simulink library "NeuroMuscularLibrary"  (R2019a)
settings: Solver=ode45  StartTime=0.0  StopTime=10.0  RelTol=1e-3  EnableMultiTasking=on
undefined symbols (not defined in the file): a2loptHAB, a2loptHAD, a2loptHAMsw, a2loptRFsw, ankle_height, aRefHAB, aRefHAD, aRefHAMsw, aRefRFsw, c, c_jointstop, deltaLegAngleThr, DeltaThRef, eref, Fmax, FmaxGLU, footBallToAnkleDist, footBallToCGDist, footBallToCGDist_y, footBallToHeelDist, footCenterlineToBall, footCenterlineToHeel, footInertia, footLength, footMass, FT, FT_GLU, GainDphiHATGLUst, GainDphiHATHABst, GainDphiHATHADst, GainDphiHATHFLst, GainFGASst, GainFGLUst, GainFHABst, GainFHAMst, GainFSOLst, GainFSOLTAst, GainFVASst, GainLBFSHst, GainLBFSHVASst, GainLGLUsw, GainLHABsw, GainLHADsw, GainLHAMGLUsw, GainLHAMsw, GainLRFHFLsw, GainLTAst, GainLTAsw, GainLVASsw, GainPhiHATGLUst, GainPhiHATHABst, GainPhiHATHADst, GainPhiHATHFLst, GainSGLUcHFLst, GainSGLUHAMst, GainSHABcHABst, GainSHADcHADst, GainSHAMBFSHsw, GainSHAMcHFLst, GainSHAMGASsw ... (+175)
libraries: sm_lib x54, $bdroot x45, nesl_utility x39, simulink x24, simulink_extras x6, vrlib x5, dspsigops x4
(part 3 of 5)

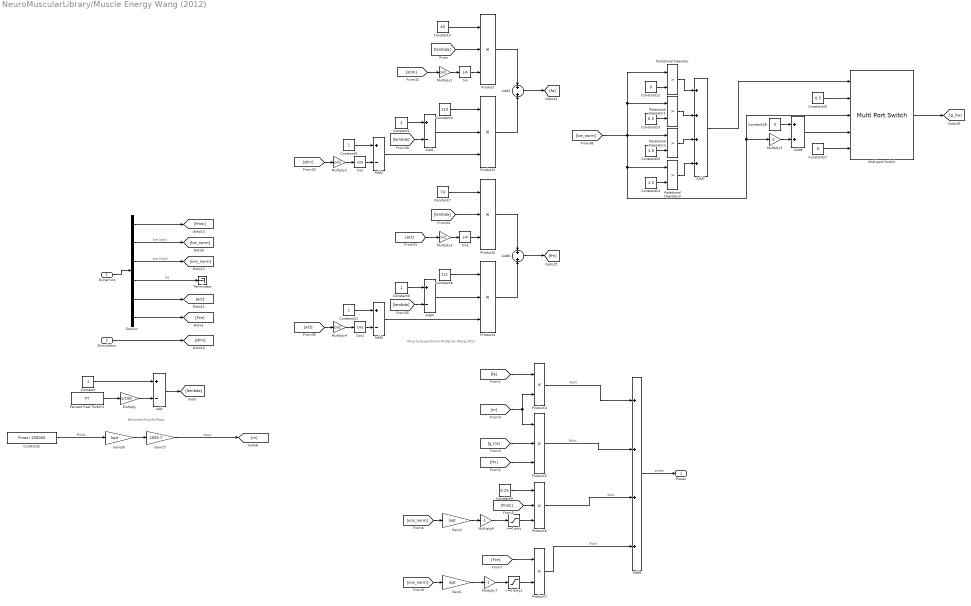
== system NeuroMuscularLibrary/Muscle Energy Wang (2012) ==
  note: Muscle Expenditure Model by Wang 2012
  note: Estimate Muscle Mass
  Dynamics : Inport
  Stimulation : Inport  Port=2
  >=0 only : Saturate  UpperLimit=inf  LowerLimit=0  ZeroCross=off
  >=0 only1 : Saturate  UpperLimit=inf  LowerLimit=0  ZeroCross=off
  Add{,1..2,4..5} (5 alike) : Sum  Inputs=+-
  Add3 : Sum
  Add6 : Sum
  Add7 : Sum  Inputs=++++
  Add8 : Sum
  Add9 : Sum  Inputs=++++
  Constant{,1,5..6,11} (5 alike) : Constant
  Constant12 : Constant  Value=0
  Constant2 : Constant  Value=Fmax/ 250000
  Constant23 : Constant  Value=0.5
  Constant24 : Constant  Value=1.5
  Constant25 : Constant  Value=1.0
  Constant26 : Constant  Value=0.5
  Constant27 : Constant  Value=0
  Constant28 : Constant  Value=3
  Constant3 : Constant  Value=40
  Constant4 : Constant  Value=133
  Constant7 : Constant  Value=74
  Constant8 : Constant  Value=111
  Constant9 : Constant  Value=0.25
  Cos : Trigonometry  Operator=cos
  Cos1 : Trigonometry  Operator=cos
  Demux : Demux  Outputs=6
  Gain1 : Gain  Gain=lopt
  Gain2 : Gain  Gain=lopt
  Gain26 : Gain  Gain=lopt
  Gain27 : Gain  Gain=1059.7
  Multiply : Gain  Gain=1/100
  Multiply{1..4} (4 alike) : Gain  Gain=pi/2
  Multiply5 : Gain  Gain=-2
  Multiply6 : Gain  Gain=-1
  Multiply7 : Gain  Gain=-1
  Multiport Switch : MultiPortSwitch  Inputs=4  DiagnosticForDefault=Warning
  Percent Fast Twitch1 : Constant  Value=FT
  Product{,1..3,5..6} (6 alike) : Product  Inputs=3
  Product4 : Product
  Product7 : Product
  Relational Operator{,1..3} (4 alike) : RelationalOperator  Operator=>  OutDataTypeStr=boolean  RndMeth=Simplest
  Sin : Trigonometry
  Sin1 : Trigonometry
  Terminator : Terminator
  Power : Outport  VectorParamsAs1DForOutWhenUnconnected=on
  wires:
  Demux/6 -> [Fce]
  [vce_norm] -> Gain1/1
  Product7/1 -> Add9/4  "Wdot"
  [Fce] -> Product7/1
  Multiply7/1 -> >=0 only1/1
  Product6/1 -> Add9/3  "Sdot"
  Multiply6/1 -> >=0 only/1
  [vce_norm] -> Gain2/1
  Constant9/1 -> Product6/1
  [Fmtc] -> Product6/2
  Product5/1 -> Add9/2  "Mdot"
  Product4/1 -> Add9/1  "Adot"
  [fm] -> Product5/3
  [g_lce] -> Product5/2
  [fa] -> Product4/1
  [m] -> Product4/2, Product5/1
  Constant2/1 -> Gain26/1  "PCSAL"
  Gain27/1 -> [m]  "Mass"
  Gain26/1 -> Gain27/1
  Multiply5/1 -> Add8/2
  Constant28/1 -> Add8/1
  Add8/1 -> Multiport Switch/4
  Constant27/1 -> Multiport Switch/5
  Constant26/1 -> Multiport Switch/2
  Add7/1 -> Multiport Switch/1
  Relational Operator3/1 -> Add7/4
  Relational Operator2/1 -> Add7/3
  Relational Operator1/1 -> Add7/2
  Relational Operator/1 -> Add7/1
  Constant24/1 -> Relational Operator3/2
  Constant25/1 -> Relational Operator2/2
  Constant23/1 -> Relational Operator1/2
  Constant12/1 -> Relational Operator/2
  [lce_norm] -> Multiport Switch/3, Multiply5/1, Relational Operator3/1, Relational Operator1/1, Relational Operator/1, Relational Operator2/1
  Constant7/1 -> Product2/1
  [act] -> Multiply3/1
  [act] -> Multiply4/1
  [lambda] -> Add4/2
  Cos1/1 -> Add5/2
  Multiply4/1 -> Cos1/1
  Add6/1 -> [fm]
  Constant8/1 -> Product3/1
  [lambda] -> Product2/2
  Add5/1 -> Product3/3
  Add4/1 -> Product3/2
  Multiply3/1 -> Sin1/1
  Constant6/1 -> Add4/1
  Sin1/1 -> Product2/3
  Product2/1 -> Add6/1
  Product3/1 -> Add6/2
  Constant11/1 -> Add5/1
  Cos/1 -> Add2/2
  Add3/1 -> [fa]
  Product/1 -> Add3/1
  Product1/1 -> Add3/2
  Multiply2/1 -> Cos/1
  [stim] -> Multiply2/1
  [stim] -> Multiply1/1
  Multiply1/1 -> Sin/1
  Sin/1 -> Product/3
  Constant5/1 -> Add2/1
  Add2/1 -> Product1/3
  Constant4/1 -> Product1/1
  Add1/1 -> Product1/2
  Constant3/1 -> Product/1
  Constant1/1 -> Add1/1
  [lambda] -> Add1/2
  [lambda] -> Product/2
  Add/1 -> [lambda]
  Multiply/1 -> Add/2
  Percent Fast Twitch1/1 -> Multiply/1
  Constant/1 -> Add/1
  Add9/1 -> Power/1  "power"
  Dynamics/1 -> Demux/1
  Stimulation/1 -> [stim]
  Demux/1 -> [Fmtc]
  Demux/3 -> [vce_norm]  "vce [lopt]"
  Demux/5 -> [act]
  Demux/4 -> Terminator/1  "lse"
  Demux/2 -> [lce_norm]  "lce [opt]"
  >=0 only/1 -> Product6/3
  >=0 only1/1 -> Product7/2
  Multiport Switch/1 -> [g_lce]
  Gain1/1 -> Multiply7/1
  Gain2/1 -> Multiply6/1

== system NeuroMuscularLibrary/Norm ==
  Vector : Inport
  Add4 : Sum  Inputs=+
  Square : Math  Operator=square  SaturateOnIntegerOverflow=on
  Square Root : Sqrt  SaturateOnIntegerOverflow=on
  Norm : Outport  VectorParamsAs1DForOutWhenUnconnected=on
  wires:
  Add4/1 -> Square Root/1
  Square/1 -> Add4/1
  Vector/1 -> Square/1
  Square Root/1 -> Norm/1

== system NeuroMuscularLibrary/Overextension Joint Limit ==
  note: Knee/Hip Joint Limits
  phi [rad] : Inport
  dphi [rad/s] : Inport  Port=2
  Gain1 : Gain  Gain=ext
  Gain2 : Gain  Gain=-ext
  Gain3 : Gain  Gain=c_jointstop
  Gain4 : Gain  Gain=1/w_max_jointstop
  Gain5 : Gain  Gain=ext
  Limit Ankle Range : simulink/Logic and Bit Operations/Interval Test  Commented=on  IntervalClosedRight=on  uplimit=185*pi/180  IntervalClosedLeft=on  lowlimit=40*pi/180  OutDataTypeStr=boolean
  Logical Operator3 : Logic  Commented=on  Operator=NOT  AllPortsSameDT=off  OutDataTypeStr=boolean
  Mux3 : Mux  Inputs=2
  Overextension Torque : Fcn  Expr="- u(1)  *  (1-u(2)) * (u(2)<1) * (u(1)>0)"
  Stop Simulation1 : Stop  Commented=on
  Sum : Sum  Inputs=|+-
  overextension angle : Constant  Value=phiUpLimit
  M_stop [Nm] : Outport  VectorParamsAs1DForOutWhenUnconnected=on
  wires:
  Gain5/1 -> M_stop [Nm]/1
  Overextension Torque/1 -> Gain5/1
  Logical Operator3/1 -> Stop Simulation1/1
  Limit Ankle Range/1 -> Logical Operator3/1
  Gain2/1 -> Mux3/2
  Gain4/1 -> Gain2/1
  Sum/1 -> Gain3/1
  phi [rad]/1 -> Limit Ankle Range/1, Sum/1
  overextension angle/1 -> Sum/2
  dphi [rad/s]/1 -> Gain4/1
  Mux3/1 -> Overextension Torque/1
  Gain3/1 -> Gain1/1
  Gain1/1 -> Mux3/1

== system NeuroMuscularLibrary/Overextension//Overflexion Joint Limit ==
  note: Overextension/Overflexion Joint Limit
  phi [rad] : Inport
  dphi [rad/s] : Inport  Port=2
  Gain1 : Gain  Gain=c_jointstop
  Gain2 : Gain  Gain=-1
  Gain3 : Gain  Gain=c_jointstop
  Gain4 : Gain  Gain=1/w_max_jointstop
  Limit Range : simulink/Logic and Bit Operations/Interval Test  Commented=on  IntervalClosedRight=on  uplimit=phi12_UpLimit + 40*pi/180  IntervalClosedLeft=on  lowlimit=phi12_LowLimit - 40*pi/180  OutDataTypeStr=boolean
  Logical Operator3 : Logic  Commented=on  Operator=NOT  AllPortsSameDT=off  OutDataTypeStr=boolean
  Mux1 : Mux  Inputs=2
  Mux3 : Mux  Inputs=2
  Overextension Torque : Fcn  Expr="- u(1)  *  (1-u(2)) * (u(2)<1) * (u(1)>0)"
  Overflexion Torque : Fcn  Expr="- u(1)  *  (1-u(2)) * (u(2)<1) * (u(1)<0)"
  Stop Simulation1 : Stop  Commented=on
  Sum : Sum  Inputs=|+-
  Sum1 : Sum  Inputs=|+-
  Sum2 : Sum
  overextension angle : Constant  Value=phiUpLimit
  overflexion angle : Constant  Value=phiLowLimit
  M_stop [Nm] : Outport  VectorParamsAs1DForOutWhenUnconnected=on
  wires:
  Mux3/1 -> Overextension Torque/1
  Gain3/1 -> Mux3/1
  dphi [rad/s]/1 -> Gain4/1
  overextension angle/1 -> Sum/2
  phi [rad]/1 -> Sum/1, Sum1/1, Limit Range/1
  Sum/1 -> Gain3/1
  Gain4/1 -> Gain2/1, Mux1/2
  Gain1/1 -> Mux1/1
  Sum1/1 -> Gain1/1
  overflexion angle/1 -> Sum1/2
  Mux1/1 -> Overflexion Torque/1
  Sum2/1 -> M_stop [Nm]/1
  Gain2/1 -> Mux3/2
  Overflexion Torque/1 -> Sum2/2
  Overextension Torque/1 -> Sum2/1
  Limit Range/1 -> Logical Operator3/1
  Logical Operator3/1 -> Stop Simulation1/1

== system NeuroMuscularLibrary/Pos//Rot Sensor ==
  Gain2 : Gain  Gain=-1
  Mux : Mux  Inputs=3
  PS-Simulink Converter : nesl_utility/PS-Simulink Converter  PhysicalDomain=network_engine_domain  SubClassName=ps_output  LeftPortType=input  RightPortType=output  PseudoPeriodic=off  Frequencies=[]  Unit=m  AffineConversion=off
  PS-Simulink Converter1 : nesl_utility/PS-Simulink Converter  PhysicalDomain=network_engine_domain  SubClassName=ps_output  LeftPortType=input  RightPortType=output  PseudoPeriodic=off  Frequencies=[]  Unit=m  AffineConversion=off
  PS-Simulink Converter2 : nesl_utility/PS-Simulink Converter  PhysicalDomain=network_engine_domain  SubClassName=ps_output  LeftPortType=input  RightPortType=output  PseudoPeriodic=off  Frequencies=[]  Unit=m  AffineConversion=off
  PS-Simulink Converter3 : nesl_utility/PS-Simulink Converter  PhysicalDomain=network_engine_domain  SubClassName=ps_output  LeftPortType=input  RightPortType=output  PseudoPeriodic=off  Frequencies=[]  Unit=rad  AffineConversion=off
  PS-Simulink Converter4 : nesl_utility/PS-Simulink Converter  PhysicalDomain=network_engine_domain  SubClassName=ps_output  LeftPortType=input  RightPortType=output  PseudoPeriodic=off  Frequencies=[]  Unit=rad  AffineConversion=off
  Position Sensor : sm_lib/Frames and Transforms/Transform Sensor  MeasurementFrame=World  SenseAngle=on  SenseAxis=on  SenseAngle1=off  SenseAngle2=off  SenseAngle3=off  SenseQ=off  SenseR=off  SenseOmegaX=off  SenseOmegaY=off  SenseOmegaZ=off  SenseOmega1=off  SenseOmega2=off  SenseOmega3=off  SenseQDot=off  SenseRDot=off  SenseAlphaX=off  SenseAlphaY=off  SenseAlphaZ=off  SenseAlpha1=off  SenseAlpha2=off  SenseAlpha3=off  SenseQDDot=off  SenseRDDot=off  SenseX=on  SenseY=on  SenseZ=on  SenseRad=off  SenseAzim=off  SenseDist=off  SenseInc=off  SenseXDot=off  SenseYDot=off  SenseZDot=off  SenseRadDot=off  SenseAzimDot=off  SenseDistDot=off  SenseIncDot=off  SenseXDDot=off  SenseYDDot=off  SenseZDDot=off  SenseRadDDot=off  SenseAzimDDot=off  SenseDistDDot=off  SenseIncDDot=off
  Product : Product
  Selector : Selector  InputPortWidth=3  IndexOptions=Index vector (dialog)  Indices=[3]  OutputSizes=1
  Sign : Signum
  F : PMIOPort  Side=Left
  B : PMIOPort  Port=2  Side=Right
  Position : Outport  VectorParamsAs1DForOutWhenUnconnected=on
  Rotation : Outport  Port=2  VectorParamsAs1DForOutWhenUnconnected=on
  wires:
  PS-Simulink Converter1/1 -> Mux/2
  PS-Simulink Converter/1 -> Mux/1
  Mux/1 -> Position/1
  PS-Simulink Converter2/1 -> Mux/3
  PS-Simulink Converter4/1 -> Selector/1
  Selector/1 -> Sign/1
  PS-Simulink Converter3/1 -> Product/1
  Sign/1 -> Product/2
  Gain2/1 -> Rotation/1
  Product/1 -> Gain2/1
  connections:
  Position Sensor/RConn1 -- F/RConn1
  PS-Simulink Converter3/LConn1 -- Position Sensor/RConn2
  B/RConn1 -- Position Sensor/LConn1
  Position Sensor/RConn4 -- PS-Simulink Converter/LConn1
  PS-Simulink Converter1/LConn1 -- Position Sensor/RConn5
  PS-Simulink Converter2/LConn1 -- Position Sensor/RConn6
  PS-Simulink Converter4/LConn1 -- Position Sensor/RConn3

== system NeuroMuscularLibrary/Position Sensor ==
  Mux : Mux  Inputs=3
  PS-Simulink Converter : nesl_utility/PS-Simulink Converter  PhysicalDomain=network_engine_domain  SubClassName=ps_output  LeftPortType=input  RightPortType=output  PseudoPeriodic=off  Frequencies=[]  Unit=m  AffineConversion=off
  PS-Simulink Converter1 : nesl_utility/PS-Simulink Converter  PhysicalDomain=network_engine_domain  SubClassName=ps_output  LeftPortType=input  RightPortType=output  PseudoPeriodic=off  Frequencies=[]  Unit=m  AffineConversion=off
  PS-Simulink Converter2 : nesl_utility/PS-Simulink Converter  PhysicalDomain=network_engine_domain  SubClassName=ps_output  LeftPortType=input  RightPortType=output  PseudoPeriodic=off  Frequencies=[]  Unit=m  AffineConversion=off
  Position Sensor : sm_lib/Frames and Transforms/Transform Sensor  MeasurementFrame=World  SenseAngle=off  SenseAxis=off  SenseAngle1=off  SenseAngle2=off  SenseAngle3=off  SenseQ=off  SenseR=off  SenseOmegaX=off  SenseOmegaY=off  SenseOmegaZ=off  SenseOmega1=off  SenseOmega2=off  SenseOmega3=off  SenseQDot=off  SenseRDot=off  SenseAlphaX=off  SenseAlphaY=off  SenseAlphaZ=off  SenseAlpha1=off  SenseAlpha2=off  SenseAlpha3=off  SenseQDDot=off  SenseRDDot=off  SenseX=on  SenseY=on  SenseZ=on  SenseRad=off  SenseAzim=off  SenseDist=off  SenseInc=off  SenseXDot=off  SenseYDot=off  SenseZDot=off  SenseRadDot=off  SenseAzimDot=off  SenseDistDot=off  SenseIncDot=off  SenseXDDot=off  SenseYDDot=off  SenseZDDot=off  SenseRadDDot=off  SenseAzimDDot=off  SenseDistDDot=off  SenseIncDDot=off
  World Frame : sm_lib/Frames and Transforms/World Frame
  Frame : PMIOPort  Side=Left
  Position : Outport  VectorParamsAs1DForOutWhenUnconnected=on
  wires:
  PS-Simulink Converter2/1 -> Mux/3
  Mux/1 -> Position/1
  PS-Simulink Converter/1 -> Mux/1
  PS-Simulink Converter1/1 -> Mux/2
  connections:
  Position Sensor/RConn4 -- PS-Simulink Converter2/LConn1
  Position Sensor/RConn2 -- PS-Simulink Converter/LConn1
  Position Sensor/RConn1 -- Frame/RConn1
  Position Sensor/RConn3 -- PS-Simulink Converter1/LConn1
  Position Sensor/LConn1 -- World Frame/RConn1

== system NeuroMuscularLibrary/Position Velocity Sensor ==
  Mux : Mux  Inputs=6
  PS-Simulink Converter : nesl_utility/PS-Simulink Converter  PhysicalDomain=network_engine_domain  SubClassName=ps_output  LeftPortType=input  RightPortType=output  PseudoPeriodic=off  Frequencies=[]  Unit=m  AffineConversion=off
  PS-Simulink Converter1 : nesl_utility/PS-Simulink Converter  PhysicalDomain=network_engine_domain  SubClassName=ps_output  LeftPortType=input  RightPortType=output  PseudoPeriodic=off  Frequencies=[]  Unit=m  AffineConversion=off
  PS-Simulink Converter2 : nesl_utility/PS-Simulink Converter  PhysicalDomain=network_engine_domain  SubClassName=ps_output  LeftPortType=input  RightPortType=output  PseudoPeriodic=off  Frequencies=[]  Unit=m  AffineConversion=off
  PS-Simulink Converter3 : nesl_utility/PS-Simulink Converter  PhysicalDomain=network_engine_domain  SubClassName=ps_output  LeftPortType=input  RightPortType=output  PseudoPeriodic=off  Frequencies=[]  Unit=m/s  AffineConversion=off
  PS-Simulink Converter4 : nesl_utility/PS-Simulink Converter  PhysicalDomain=network_engine_domain  SubClassName=ps_output  LeftPortType=input  RightPortType=output  PseudoPeriodic=off  Frequencies=[]  Unit=m/s  AffineConversion=off
  PS-Simulink Converter5 : nesl_utility/PS-Simulink Converter  PhysicalDomain=network_engine_domain  SubClassName=ps_output  LeftPortType=input  RightPortType=output  PseudoPeriodic=off  Frequencies=[]  Unit=m/s  AffineConversion=off
  Position Sensor : sm_lib/Frames and Transforms/Transform Sensor  MeasurementFrame=World  SenseAngle=off  SenseAxis=off  SenseAngle1=off  SenseAngle2=off  SenseAngle3=off  SenseQ=off  SenseR=off  SenseOmegaX=off  SenseOmegaY=off  SenseOmegaZ=off  SenseOmega1=off  SenseOmega2=off  SenseOmega3=off  SenseQDot=off  SenseRDot=off  SenseAlphaX=off  SenseAlphaY=off  SenseAlphaZ=off  SenseAlpha1=off  SenseAlpha2=off  SenseAlpha3=off  SenseQDDot=off  SenseRDDot=off  SenseX=on  SenseY=on  SenseZ=on  SenseRad=off  SenseAzim=off  SenseDist=off  SenseInc=off  SenseXDot=on  SenseYDot=on  SenseZDot=on  SenseRadDot=off  SenseAzimDot=off  SenseDistDot=off  SenseIncDot=off  SenseXDDot=off  SenseYDDot=off  SenseZDDot=off  SenseRadDDot=off  SenseAzimDDot=off  SenseDistDDot=off  SenseIncDDot=off
  World Frame1 : sm_lib/Frames and Transforms/World Frame
  Frame : PMIOPort  Side=Left
  Position and Velocity : Outport  VectorParamsAs1DForOutWhenUnconnected=on
  wires:
  PS-Simulink Converter1/1 -> Mux/2
  PS-Simulink Converter/1 -> Mux/1
  Mux/1 -> Position and Velocity/1
  PS-Simulink Converter2/1 -> Mux/3
  PS-Simulink Converter3/1 -> Mux/4
  PS-Simulink Converter4/1 -> Mux/5
  PS-Simulink Converter5/1 -> Mux/6
  connections:
  Position Sensor/RConn3 -- PS-Simulink Converter1/LConn1
  Position Sensor/RConn1 -- Frame/RConn1
  Position Sensor/RConn2 -- PS-Simulink Converter/LConn1
  Position Sensor/RConn4 -- PS-Simulink Converter2/LConn1
  Position Sensor/LConn1 -- World Frame1/RConn1
  PS-Simulink Converter3/LConn1 -- Position Sensor/RConn5
  PS-Simulink Converter4/LConn1 -- Position Sensor/RConn6
  PS-Simulink Converter5/LConn1 -- Position Sensor/RConn7

== system NeuroMuscularLibrary/RF Link ==
  note: RF Attachment
  hip angle : Inport
  knee angle : Inport  Port=2
  Constant3 : Constant  Value=rRFh
  Constant4 : Constant  Value=lslackRF+loptRF
  Constant5 : Constant  Value=phirefRFh
  Constant6 : Constant  Value=phirefRFk
  Constant7 : Constant  Value=phimaxRFk  VectorParams1D=off
  Demux1 : Demux  Outputs=2
  Gain1 : Gain  Gain=phiScaleRFk
  Gain2 : Gain  Gain=rhoRFh
  Gain3 : Gain  Gain=rRFkmax
  Gain4 : Gain  Gain=rhoRFk/phiScaleRFk
  Gain5 : Gain  Gain=phiScaleRFk
  Mux1 : Mux  Inputs=2
  Product : Product  RndMeth=Zero
  Sum4 : Sum  Inputs=|+-
  Sum5 : Sum  Inputs=+++
  Sum7 : Sum  Inputs=|+-
  Sum8 : Sum  Inputs=-+|
  Sum9 : Sum  Inputs=-+
  length change term ankle : Trigonometry
  offset correction term ankle : Trigonometry
  variable lever term ankle : Trigonometry  Operator=cos
  lmtu [m] : Outport  VectorParamsAs1DForOutWhenUnconnected=on
  hip lever [m] : Outport  Port=2  VectorParamsAs1DForOutWhenUnconnected=on
  knee lever [m] : Outport  Port=3  VectorParamsAs1DForOutWhenUnconnected=on
  wires:
  Gain2/1 -> Sum5/1
  Gain4/1 -> Sum5/3
  Gain3/1 -> Demux1/1
  Mux1/1 -> Gain3/1
  Constant4/1 -> Sum5/2
  Sum9/1 -> Mux1/1
  offset correction term ankle/1 -> Sum9/1
  length change term ankle/1 -> Sum9/2
  Constant6/1 -> Sum7/1
  Sum7/1 -> Gain1/1
  Constant7/1 -> Sum7/2, Sum8/1
  Sum8/1 -> Gain5/1
  Demux1/2 -> knee lever [m]/1
  variable lever term ankle/1 -> Mux1/2
  Sum5/1 -> lmtu [m]/1
  Product/1 -> Gain2/1
  Constant3/1 -> Product/2, hip lever [m]/1
  Sum4/1 -> Product/1
  Constant5/1 -> Sum4/2
  Gain5/1 -> length change term ankle/1, variable lever term ankle/1
  Gain1/1 -> offset correction term ankle/1
  knee angle/1 -> Sum8/2
  hip angle/1 -> Sum4/1
  Demux1/1 -> Gain4/1

== system NeuroMuscularLibrary/RF amp Link ==
  note: RF Attachment
  hip angle : Inport
  Constant3 : Constant  Value=rRFh
  Constant4 : Constant  Value=lslackRFamp+loptRFamp
  Constant5 : Constant  Value=phirefRFh
  Gain2 : Gain  Gain=rhoRFh
  Product : Product  RndMeth=Zero
  Sum4 : Sum  Inputs=|+-
  Sum5 : Sum
  lmtu [m] : Outport  VectorParamsAs1DForOutWhenUnconnected=on
  hip lever [m] : Outport  Port=2  VectorParamsAs1DForOutWhenUnconnected=on
  wires:
  hip angle/1 -> Sum4/1
  Constant5/1 -> Sum4/2
  Sum4/1 -> Product/1
  Constant3/1 -> hip lever [m]/1, Product/2
  Product/1 -> Gain2/1
  Sum5/1 -> lmtu [m]/1
  Constant4/1 -> Sum5/2
  Gain2/1 -> Sum5/1

== system NeuroMuscularLibrary/Rotational Position Velocity Sensor ==
  Demux : Demux  Outputs=3
  Mux : Mux  Inputs=6
  PS-Simulink Converter{,1,3..5} (5 alike) : nesl_utility/PS-Simulink Converter  PhysicalDomain=network_engine_domain  SubClassName=ps_output  LeftPortType=input  RightPortType=output  PseudoPeriodic=off  Frequencies=[]  Unit=inherit  AffineConversion=off
  Position Sensor : sm_lib/Frames and Transforms/Transform Sensor  MeasurementFrame=World  SenseAngle=on  SenseAxis=on  SenseAngle1=off  SenseAngle2=off  SenseAngle3=off  SenseQ=off  SenseR=off  SenseOmegaX=on  SenseOmegaY=on  SenseOmegaZ=on  SenseOmega1=off  SenseOmega2=off  SenseOmega3=off  SenseQDot=off  SenseRDot=off  SenseAlphaX=off  SenseAlphaY=off  SenseAlphaZ=off  SenseAlpha1=off  SenseAlpha2=off  SenseAlpha3=off  SenseQDDot=off  SenseRDDot=off  SenseX=off  SenseY=off  SenseZ=off  SenseRad=off  SenseAzim=off  SenseDist=off  SenseInc=off  SenseXDot=off  SenseYDot=off  SenseZDot=off  SenseRadDot=off  SenseAzimDot=off  SenseDistDot=off  SenseIncDot=off  SenseXDDot=off  SenseYDDot=off  SenseZDDot=off  SenseRadDDot=off  SenseAzimDDot=off  SenseDistDDot=off  SenseIncDDot=off
  Product : Product
  World Frame1 : sm_lib/Frames and Transforms/World Frame
  Frame : PMIOPort  Side=Left
  Position and Velocity : Outport  VectorParamsAs1DForOutWhenUnconnected=on
  wires:
  PS-Simulink Converter5/1 -> Mux/6
  PS-Simulink Converter4/1 -> Mux/5
  PS-Simulink Converter3/1 -> Mux/4
  Demux/3 -> Mux/3
  Mux/1 -> Position and Velocity/1
  PS-Simulink Converter/1 -> Product/1
  PS-Simulink Converter1/1 -> Product/2
  Product/1 -> Demux/1
  Demux/2 -> Mux/2
  Demux/1 -> Mux/1
  connections:
  PS-Simulink Converter5/LConn1 -- Position Sensor/RConn6
  PS-Simulink Converter4/LConn1 -- Position Sensor/RConn5
  Position Sensor/LConn1 -- World Frame1/RConn1
  Position Sensor/RConn4 -- PS-Simulink Converter3/LConn1
  Position Sensor/RConn2 -- PS-Simulink Converter/LConn1
  Position Sensor/RConn1 -- Frame/RConn1
  Position Sensor/RConn3 -- PS-Simulink Converter1/LConn1

== system NeuroMuscularLibrary/SOL Link ==
  note: Soleus Attachment
  Ankle angle [rad] : Inport
  Constant : Constant  Value=lslackSOL+loptSOL
  Constant3 : Constant  Value=phimaxSOL
  Constant5 : Constant  Value=phirefSOL
  Demux1 : Demux  Outputs=2
  Gain2 : Gain  Gain=rSOLmax
  Gain3 : Gain  Gain=phiScaleSOL
  Gain8 : Gain  Gain=phiScaleSOL
  Gain9 : Gain  Gain=rhoSOL/phiScaleSOL
  Mux1 : Mux  Inputs=2
  Sum4 : Sum  Inputs=-+
  Sum5 : Sum  Inputs=|+-
  Sum6 : Sum  Inputs=|+-
  Sum7 : Sum  Inputs=-+|
  length change term : Trigonometry
  offset correction term : Trigonometry
  variable lever term : Trigonometry  Operator=cos
  lmtc [m] : Outport  VectorParamsAs1DForOutWhenUnconnected=on
  lever [m] : Outport  Port=2  VectorParamsAs1DForOutWhenUnconnected=on
  wires:
  Gain8/1 -> offset correction term/1
  Gain3/1 -> variable lever term/1, length change term/1
  length change term/1 -> Sum4/2
  offset correction term/1 -> Sum4/1
  Mux1/1 -> Gain2/1
  Gain2/1 -> Demux1/1
  Sum4/1 -> Mux1/1
  variable lever term/1 -> Mux1/2
  Constant3/1 -> Sum7/1, Sum6/2
  Constant/1 -> Sum5/1
  Sum7/1 -> Gain3/1
  Constant5/1 -> Sum6/1
  Sum6/1 -> Gain8/1
  Gain9/1 -> Sum5/2
  Demux1/2 -> lever [m]/1
  Demux1/1 -> Gain9/1
  Sum5/1 -> lmtc [m]/1
  Ankle angle [rad]/1 -> Sum7/2

== system NeuroMuscularLibrary/Self collision detector ==
  Left hip PosVel : Inport
  Left knee pos : Inport  Port=2
  Left ankle pos : Inport  Port=3
  Right hip PosVel : Inport  Port=4
  Right knee pos : Inport  Port=5
  Right ankle pos : Inport  Port=6
  Past init steps? : Inport  Port=7
  Cast To Double : DataTypeConversion  OutDataTypeStr=double
  Cast To Double1 : DataTypeConversion  OutDataTypeStr=double
  Compare To Constant : simulink/Logic and Bit Operations/Compare To Constant  relop=<=  const=maxDist  OutDataTypeStr=uint8
  Distance between Lthigh Rshank : $bdroot/Distance between lines  SystemSampleTime=-1  Latency=0  AutoFrameSizeCalculation=off
  Distance between Rthigh Lshank : $bdroot/Distance between lines  SystemSampleTime=-1  Latency=0  AutoFrameSizeCalculation=off
  Distance between shanks : $bdroot/Distance between lines  SystemSampleTime=-1  Latency=0  AutoFrameSizeCalculation=off
  Distance between thighs : $bdroot/Distance between lines  SystemSampleTime=-1  Latency=0  AutoFrameSizeCalculation=off
  Max : MinMax  Function=max
  Mux{,1..3} (4 alike) : Mux  Inputs=[3 3]
  Mux4 : Mux
  Product : Product
  Selector : Selector  InputPortWidth=6  IndexOptions=Index vector (dialog)  Indices=[1 2 3]  OutputSizes=1
  Selector1 : Selector  InputPortWidth=6  IndexOptions=Index vector (dialog)  Indices=[1 2 3]  OutputSizes=1
  Distances : Outport  VectorParamsAs1DForOutWhenUnconnected=on
  Limb contact? : Outport  Port=2  VectorParamsAs1DForOutWhenUnconnected=on
  wires:
  Left hip PosVel/1 -> Selector/1
  Left knee pos/1 -> Mux1/1, Mux/2
  Left ankle pos/1 -> Mux1/2
  Mux/1 -> [Lthigh]
  Mux1/1 -> [Lshank]
  Right hip PosVel/1 -> Selector1/1
  Mux3/1 -> [Rshank]
  Right knee pos/1 -> Mux2/2, Mux3/1
  Right ankle pos/1 -> Mux3/2
  Mux2/1 -> [Rthigh]
  [Lthigh] -> Distance between thighs/1
  [Rthigh] -> Distance between thighs/2
  [Rshank] -> Distance between shanks/2
  [Lshank] -> Distance between shanks/1
  [Lthigh] -> Distance between Lthigh Rshank/1
  [Rshank] -> Distance between Lthigh Rshank/2
  [Lshank] -> Distance between Rthigh Lshank/2
  [Rthigh] -> Distance between Rthigh Lshank/1
  Distance between thighs/1 -> Mux4/1
  Distance between Lthigh Rshank/1 -> Mux4/2
  Distance between Rthigh Lshank/1 -> Mux4/3
  Distance between shanks/1 -> Mux4/4
  Mux4/1 -> Cast To Double/1
  Compare To Constant/1 -> Max/1
  Max/1 -> Cast To Double1/1
  Selector/1 -> Mux/1
  Selector1/1 -> Mux2/1
  Cast To Double/1 -> Distances/1, Compare To Constant/1
  Cast To Double1/1 -> Product/1
  Product/1 -> Limb contact?/1
  Past init steps?/1 -> Product/2

== system NeuroMuscularLibrary/Sensor Sheet ==
  note: Inner Segment Pressure Sheet
  FB Gain1 : Gain  Gain=1/DeltaThRef  SaturateOnIntegerOverflow=on  OutDataTypeStr=Inherit: Same as input  ParamDataTypeStr=Inherit: Same as input
  Gain1 : Gain  Gain=-1
  Gain3 : Gain  Gain=k_pressure
  Gain4 : Gain  Gain=1/v_max_pressure
  Mux1 : Mux  Inputs=2
  PS-Simulink Converter : nesl_utility/PS-Simulink Converter  PhysicalDomain=network_engine_domain  SubClassName=ps_output  LeftPortType=input  RightPortType=output  PseudoPeriodic=off  Frequencies=[]  Unit=1  AffineConversion=off
  PS-Simulink Converter1 : nesl_utility/PS-Simulink Converter  PhysicalDomain=network_engine_domain  SubClassName=ps_output  LeftPortType=input  RightPortType=output  PseudoPeriodic=off  Frequencies=[]  Unit=1  AffineConversion=off
  Pressure Sheet Reaction Force : Fcn  Expr=-u(1) * (1+sgn(u(1))*u(2))
  Prismatic Joint : sm_lib/Joints/Prismatic Joint  SenseConstraintForce=off  SenseConstraintForceX=off  SenseConstraintForceY=off  SenseConstraintForceZ=off  SenseConstraintTorque=off  SenseConstraintTorqueX=off  SenseConstraintTorqueY=off  SenseConstraintTorqueZ=off  SenseTotalForce=off  SenseTotalForceX=off  SenseTotalForceY=off  SenseTotalForceZ=off  SenseTotalTorque=off  SenseTotalTorqueX=off  SenseTotalTorqueY=off  SenseTotalTorqueZ=off  CompositeWrenchDir=FollowerOnBase  CompositeWrenchFrame=BaseFrame  EquilibriumPosition=0  EquilibriumPositionUnits=m  SpringStiffness=0  SpringStiffnessUnits=N/m  DampingCoefficient=0  DampingCoefficientUnits=N/(m/s)  TorqueActuationMode=InputTorque  MotionActuationMode=ComputedMotion  SensePosition=on  SenseVelocity=on  SenseAcceleration=off  SenseTorqueForce=off  SenseLowerLimitTorqueForce=off  SenseUpperLimitTorqueForce=off  LowerLimitSpecify=off  LowerLimitBound=-1  LowerLimitBoundUnits=m  LowerLimitStiffness=1e6  LowerLimitStiffnessUnits=N/m  LowerLimitDamping=1e3  LowerLimitDampingUnits=N/(m/s)  LowerLimitTransitionRegionWidth=1e-4  LowerLimitTransitionRegionWidthUnits=m  UpperLimitSpecify=off  UpperLimitBound=1  UpperLimitBoundUnits=m  UpperLimitStiffness=1e6  UpperLimitStiffnessUnits=N/m  UpperLimitDamping=1e3  UpperLimitDampingUnits=N/(m/s)  UpperLimitTransitionRegionWidth=1e-4  UpperLimitTransitionRegionWidthUnits=m  PositionTargetSpecify=on  PositionTargetPriority=High  PositionTargetValue=0  PositionTargetValueUnits=m  VelocityTargetSpecify=on  VelocityTargetPriority=High  VelocityTargetValue=0  VelocityTargetValueUnits=m/s
  Saturation11 : Saturate  UpperLimit=inf  LowerLimit=0  ZeroCross=off
  Simulink-PS Converter : nesl_utility/Simulink-PS Converter  PhysicalDomain=network_engine_domain  SubClassName=ps_input  LeftPortType=input  RightPortType=output  PseudoPeriodic=off  Frequencies=[]  NoiseDistribution=none  NoiseParameters=[]  Unit=1  AffineConversion=off  FilteringAndDerivatives=zero  SimscapeFilterOrder=1  InputFilterTimeConstant=0.001  UdotUserProvided=1
  Y-up TO Z-up : sm_lib/Frames and Transforms/Rigid Transform  TranslationMethod=None  TranslationStandardOffset=0  TranslationLengthUnit=m  TranslationStandardAxis=+Z  TranslationCartesianOffset=[0 0 0]  TranslationROffset=0  TranslationROffsetUnits=m  TranslationZOffset=0  TranslationZOffsetUnits=m  TranslationThetaOffset=0  TranslationThetaOffsetUnits=deg  RotationMethod=AlignedAxes  RotationAngleUnits=deg  RotationStandardAxis=+Z  RotationAngle=0  RotationArbitraryAxis=[0 0 1]  FollAlignAxisA=+X  BaseAlignAxisA=+X  FollAlignAxisB=+Z  BaseAlignAxisB=+Y  RotationSequenceAxes=FollowerAxes  RotationSequence=XYX  RotationSequenceAngles=[0 0 0]  RotationSequenceAnglesUnits=deg  RotationMatrix=[1 0 0; 0 1 0; 0 0 1]
  Z-up TO Y-up : sm_lib/Frames and Transforms/Rigid Transform  TranslationMethod=None  TranslationStandardOffset=0  TranslationLengthUnit=m  TranslationStandardAxis=+Z  TranslationCartesianOffset=[0 0 0]  TranslationROffset=0  TranslationROffsetUnits=m  TranslationZOffset=0  TranslationZOffsetUnits=m  TranslationThetaOffset=0  TranslationThetaOffsetUnits=deg  RotationMethod=AlignedAxes  RotationAngleUnits=deg  RotationStandardAxis=+Z  RotationAngle=0  RotationArbitraryAxis=[0 0 1]  FollAlignAxisA=+X  BaseAlignAxisA=+X  FollAlignAxisB=+Y  BaseAlignAxisB=+Z  RotationSequenceAxes=FollowerAxes  RotationSequence=XYX  RotationSequenceAngles=[0 0 0]  RotationSequenceAnglesUnits=deg  RotationMatrix=[1 0 0; 0 1 0; 0 0 1]
  smooth : TransferFcn  Denominator=[0.02 1]
  Thigh : PMIOPort  Side=Left
  Hip Joint : PMIOPort  Port=2  Side=Right
  dx : Outport  VectorParamsAs1DForOutWhenUnconnected=on
  Thigh Fx : Outport  Port=2  VectorParamsAs1DForOutWhenUnconnected=on
  wires:
  PS-Simulink Converter/1 -> Gain1/1, Gain3/1  "position"
  PS-Simulink Converter1/1 -> Gain4/1  "velocity"
  Mux1/1 -> Pressure Sheet Reaction Force/1
  Gain3/1 -> Mux1/1
  Gain4/1 -> Mux1/2
  Pressure Sheet Reaction Force/1 -> Simulink-PS Converter/1
  FB Gain1/1 -> Thigh Fx/1
  smooth/1 -> Saturation11/1
  Saturation11/1 -> FB Gain1/1
  Gain1/1 -> smooth/1, dx/1
  connections:
  Prismatic Joint/LConn1 -- Y-up TO Z-up/RConn1
  Prismatic Joint/RConn1 -- Z-up TO Y-up/LConn1
  Prismatic Joint/LConn2 -- Simulink-PS Converter/RConn1
  Prismatic Joint/RConn2 -- PS-Simulink Converter/LConn1
  Prismatic Joint/RConn3 -- PS-Simulink Converter1/LConn1
  Y-up TO Z-up/LConn1 -- Thigh/RConn1
  Hip Joint/RConn1 -- Z-up TO Y-up/RConn1

== system NeuroMuscularLibrary/Shanks ==
  Ankle to Knee : sm_lib/Frames and Transforms/Rigid Transform  TranslationMethod=Cartesian  TranslationStandardOffset=0  TranslationLengthUnit=m  TranslationStandardAxis=+Z  TranslationCartesianOffset=[shankLength 0 0]  TranslationROffset=0  TranslationROffsetUnits=m  TranslationZOffset=0  TranslationZOffsetUnits=m  TranslationThetaOffset=0  TranslationThetaOffsetUnits=deg  RotationMethod=AlignedAxes  RotationAngleUnits=deg  RotationStandardAxis=+Z  RotationAngle=0.0  RotationArbitraryAxis=[0 0 1]  FollAlignAxisA=+Z  BaseAlignAxisA=+Z  FollAlignAxisB=+X  BaseAlignAxisB=-X  RotationSequenceAxes=FollowerAxes  RotationSequence=XYX  RotationSequenceAngles=[0 0 0]  RotationSequenceAnglesUnits=deg  RotationMatrix=[1 0 0; 0 1 0; 0 0 1]
  Cylindrical Solid : sm_lib/Body Elements/Solid  InertiaType=CalculateFromGeometry  Mass=0  MassUnits=kg  CenterOfMass=[0 0 0]  CenterOfMassUnits=m  MomentsOfInertia=[1 1 1]  MomentsOfInertiaUnits=kg*m^2  ProductsOfInertia=[0 0 0]  ProductsOfInertiaUnits=kg*m^2  BasedOnType=Mass  Density=0  DensityUnits=kg/m^3  DoExposeReferenceFrame=on  SerializedFrames=<Frames/>  GraphicType=FromGeometry  MarkerShape=Sphere  MarkerSize=10  GraphicVisPropType=SimpleVisualProperties  GraphicDiffuseColor=[0.5 0.5 0.5]  GraphicSpecularColor=[0.5 0.5 0.5 1.0]  GraphicAmbientColor=[0.15 0.15 0.15 1.0]  GraphicEmissiveColor=[0.0 0.0 0.0 1.0]  GraphicShininess=75  GraphicOpacity=1.0  GeometryShape=Cylinder  RectangleSize=[1 1]  RectangleSizeUnits=m  BrickDimensions=[1 1 1]  BrickDimensionUnits=m  CylinderRadius=.04  CylinderRadiusUnits=m  CylinderLength=shankLength  CylinderLengthUnits=m  SphereRadius=1  SphereRadiusUnits=m  EllipsoidRadii=[1 1 1]  EllipsoidRadiiUnits=m  ExtrusionCrossSection=[1 1; -1 1; -1 -1; 1 -1]  ExtrusionCrossSectionUnits=m  ExtrusionLength=1  ExtrusionLengthUnits=m  PolygonNumSides=3  PolygonOuterRadius=1  PolygonOuterRadiusUnits=m  ExtGeomFileType=STEP  ExtGeomFileUnits=m  RevolutionCrossSection=[1 1; 1 -1; 2 -1; 2 1]  RevolutionCrossSectionUnits=m  RevolutionExtent=Full  RevolutionAngle=180  RevolutionAngleUnits=deg
  Inertia : sm_lib/Body Elements/Inertia  InertiaType=Custom  Mass=shankMass  MassUnits=kg  CenterOfMass=[0 0 0]  CenterOfMassUnits=m  MomentsOfInertia=shankInertia  MomentsOfInertiaUnits=kg*m^2  ProductsOfInertia=[0 0 0]  ProductsOfInertiaUnits=kg*m^2  GraphicType=None  MarkerShape=Inertia  MarkerSize=20  GraphicVisPropType=SimpleVisualProperties  GraphicDiffuseColor=[0.5 0.5 0.5]  GraphicSpecularColor=[0.5 0.5 0.5 1.0]  GraphicAmbientColor=[0.15 0.15 0.15 1.0]  GraphicEmissiveColor=[0.0 0.0 0.0 1.0]  GraphicShininess=75  GraphicOpacity=1.0
  To CG : sm_lib/Frames and Transforms/Rigid Transform  TranslationMethod=Cartesian  TranslationStandardOffset=0  TranslationLengthUnit=m  TranslationStandardAxis=+Z  TranslationCartesianOffset=[shankAnkleToCGDist 0 0]  TranslationROffset=0  TranslationROffsetUnits=m  TranslationZOffset=0  TranslationZOffsetUnits=m  TranslationThetaOffset=0  TranslationThetaOffsetUnits=deg  RotationMethod=AlignedAxes  RotationAngleUnits=deg  RotationStandardAxis=+Z  RotationAngle=0.0  RotationArbitraryAxis=[0 0 1]  FollAlignAxisA=+Z  BaseAlignAxisA=+X  FollAlignAxisB=+X  BaseAlignAxisB=-Y  RotationSequenceAxes=FollowerAxes  RotationSequence=XYX  RotationSequenceAngles=[0 0 0]  RotationSequenceAnglesUnits=deg  RotationMatrix=[1 0 0; 0 1 0; 0 0 1]
  To center : sm_lib/Frames and Transforms/Rigid Transform  TranslationMethod=Cartesian  TranslationStandardOffset=0  TranslationLengthUnit=m  TranslationStandardAxis=+Z  TranslationCartesianOffset=[shankLength/2 0 0]  TranslationROffset=0  TranslationROffsetUnits=m  TranslationZOffset=0  TranslationZOffsetUnits=m  TranslationThetaOffset=0  TranslationThetaOffsetUnits=deg  RotationMethod=AlignedAxes  RotationAngleUnits=deg  RotationStandardAxis=+Z  RotationAngle=0.0  RotationArbitraryAxis=[0 0 1]  FollAlignAxisA=+Z  BaseAlignAxisA=+X  FollAlignAxisB=+Y  BaseAlignAxisB=+Y  RotationSequenceAxes=FollowerAxes  RotationSequence=XYX  RotationSequenceAngles=[0 0 0]  RotationSequenceAnglesUnits=deg  RotationMatrix=[1 0 0; 0 1 0; 0 0 1]
  "X-up, Y-back Z-lateral to X-down, Y-front, Z-medial " : sm_lib/Frames and Transforms/Rigid Transform  Commented=on  TranslationMethod=None  TranslationStandardOffset=0  TranslationLengthUnit=m  TranslationStandardAxis=+Z  TranslationCartesianOffset=[0 0 0]  TranslationROffset=0  TranslationROffsetUnits=m  TranslationZOffset=0  TranslationZOffsetUnits=m  TranslationThetaOffset=0  TranslationThetaOffsetUnits=deg  RotationMethod=AlignedAxes  RotationAngleUnits=deg  RotationStandardAxis=+Z  RotationAngle=0.0  RotationArbitraryAxis=[0 0 1]  FollAlignAxisA=+Z  BaseAlignAxisA=+Z  FollAlignAxisB=+X  BaseAlignAxisB=-X  RotationSequenceAxes=FollowerAxes  RotationSequence=XYX  RotationSequenceAngles=[0 0 0]  RotationSequenceAnglesUnits=deg  RotationMatrix=[1 0 0; 0 1 0; 0 0 1]
  CG : PMIOPort  Side=Right
  Ankle : PMIOPort  Port=2  Side=Right
  Knee : PMIOPort  Port=3  Side=Left
  connections:
  To CG/LConn1 -- Ankle/RConn1 -- Ankle to Knee/LConn1 -- To center/LConn1
  To CG/RConn1 -- CG/RConn1 -- Inertia/RConn1
  Knee/RConn1 -- Ankle to Knee/RConn1
  To center/RConn1 -- Cylindrical Solid/RConn1

== system NeuroMuscularLibrary/Stance Phase (coronal) ==
  note: Stance Phase Control
  note: M3: balance trunk
  note: M4: compensate swing leg
  thetaHATref : Inport
  theta dtheta HAT [rad rad/s] : Inport  Port=2
  CSwingStim : Inport  Port=3
  FmHAB : Inport  Port=4
  Enable : EnablePort  StatesWhenEnabling=reset  ZeroCross=off
  " 1" : Gain  Gain=GainPhiHATHABst
  " 2" : Gain  Gain=GainDphiHATHABst
  " 3" : Gain  Gain=GainFHABst
  " 4" : Gain  Gain=GainPhiHATHADst
  " 5" : Gain  Gain=GainDphiHATHADst
  " 6" : Gain  Gain=GainSHABcHABst
  " 7" : Gain  Gain=GainSHADcHADst
  Constant12 : Constant  Value=PreStimHADst
  Constant15 : Constant  Value=PreStimHABst
  Demux7 : Demux  Outputs=2
  Demux8 : Demux  Outputs=2
  Gain2 : Gain  Gain=-1
  Gain3 : Gain  Gain=-1
  Mux : Mux  Inputs=2
  Mux1 : Mux  Inputs=2
  Mux2 : Mux  Inputs=2
  Sum4 : Sum  Inputs=-+|  SaturateOnIntegerOverflow=on  InputSameDT=on  OutDataTypeStr=Inherit: Same as first input
  Sum5 : Sum  SaturateOnIntegerOverflow=on  InputSameDT=on  OutDataTypeStr=Inherit: Same as first input
  Sum6 : Sum  SaturateOnIntegerOverflow=on  InputSameDT=on  OutDataTypeStr=Inherit: Same as first input
  positive half1 : Saturate  UpperLimit=inf  LowerLimit=0  ZeroCross=off
  positive half2 : Saturate  UpperLimit=inf  LowerLimit=0  ZeroCross=off
  S_0_St : Outport  OutputWhenDisabled=reset  InitialOutput=0  VectorParamsAs1DForOutWhenUnconnected=on
  S_M1 [HAB] : Outport  Port=2  OutputWhenDisabled=reset  InitialOutput=0  VectorParamsAs1DForOutWhenUnconnected=on
  S_M3 [HAB HAD] : Outport  Port=3  OutputWhenDisabled=reset  InitialOutput=0  VectorParamsAs1DForOutWhenUnconnected=on
  S_M4 [HAB HAD] : Outport  Port=4  OutputWhenDisabled=reset  InitialOutput=0  VectorParamsAs1DForOutWhenUnconnected=on
  wires:
  theta dtheta HAT [rad rad/s]/1 -> Demux7/1
  Demux7/1 -> Sum4/2  "theta"
  Demux7/2 -> " 5"/1, Gain3/1  "dtheta"
  thetaHATref/1 -> Sum4/1
  Sum4/1 -> " 4"/1, Gain2/1
  Gain2/1 -> " 1"/1
  Gain3/1 -> " 2"/1
  " 1"/1 -> Sum5/1
  " 2"/1 -> Sum5/2
  " 4"/1 -> Sum6/1
  " 5"/1 -> Sum6/2
  Sum5/1 -> positive half1/1  "HAB"
  Sum6/1 -> positive half2/1  "HAD"
  Mux1/1 -> S_M3 [HAB HAD]/1
  Mux/1 -> S_0_St/1
  CSwingStim/1 -> Demux8/1
  Mux2/1 -> S_M4 [HAB HAD]/1
  Demux8/1 -> " 6"/1  "Stim_CHAB"
  Demux8/2 -> " 7"/1  "Stim_CHAD"
  " 6"/1 -> Mux2/1  "HAB"
  " 7"/1 -> Mux2/2  "HAD"
  positive half1/1 -> Mux1/1
  positive half2/1 -> Mux1/2
  " 3"/1 -> S_M1 [HAB]/1  "HAB"
  FmHAB/1 -> " 3"/1
  Constant12/1 -> Mux/2
  Constant15/1 -> Mux/1

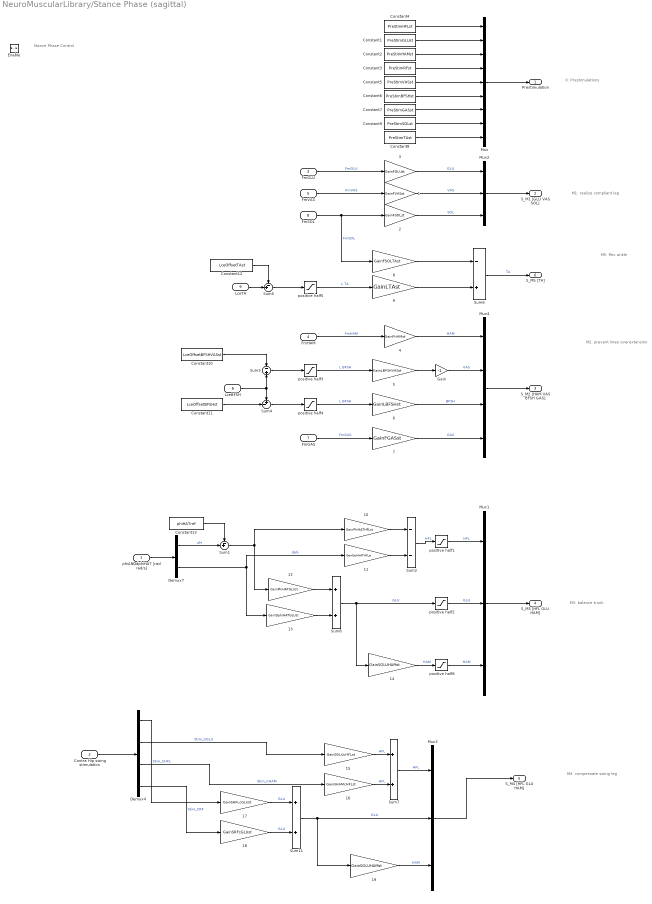
== system NeuroMuscularLibrary/Stance Phase (sagittal) ==
  note: M4: compensate swing leg
  note: M3: balance trunk
  note: M5: flex ankle
  note: M2: prevent knee overextension
  note: M1: realize compliant leg
  note: 0: Prestimulations
  note: Stance Phase Control
  phiANDdphiHAT [rad rad/s] : Inport
  Contra Hip swing stimulation : Inport  Port=2
  FmGLU : Inport  Port=3
  FmHAM : Inport  Port=4
  FmVAS : Inport  Port=5
  LceBFSH : Inport  Port=6
  FmGAS : Inport  Port=7
  FmSOL : Inport  Port=8
  LceTA : Inport  Port=9
  Enable : EnablePort  StatesWhenEnabling=reset  ZeroCross=off
  " 1" : Gain  Gain=GainFVASst
  " 10" : Gain  Gain=GainPhiHATHFLst
  " 11" : Gain  Gain=GainDphiHATHFLst
  " 12" : Gain  Gain=GainPhiHATGLUst
  " 13" : Gain  Gain=GainDphiHATGLUst
  " 14" : Gain  Gain=GainSGLUHAMst
  " 15" : Gain  Gain=GainSGLUcHFLst
  " 16" : Gain  Gain=GainSHAMcHFLst
  " 17" : Gain  Gain=GainSHFLcGLUst
  " 18" : Gain  Gain=GainSRFcGLUst
  " 19" : Gain  Gain=GainSGLUHAMst
  " 2" : Gain  Gain=GainFSOLst
  " 3" : Gain  Gain=GainFGLUst
  " 4" : Gain  Gain=GainFHAMst
  " 5" : Gain  Gain=GainLBFSHVASst
  " 6" : Gain  Gain=GainLBFSHst
  " 7" : Gain  Gain=GainFGASst
  " 8" : Gain  Gain=GainFSOLTAst
  " 9" : Gain  Gain=GainLTAst
  Constant1 : Constant  Value=PreStimGLUst
  Constant10 : Constant  Value=LceOffsetBFSHVASst
  Constant11 : Constant  Value=LceOffsetBFSHst
  Constant12 : Constant  Value=LceOffsetTAst
  Constant13 : Constant  Value=phiHATref
  Constant2 : Constant  Value=PreStimHAMst
  Constant3 : Constant  Value=PreStimRFst
  Constant4 : Constant  Value=PreStimHFLst
  Constant5 : Constant  Value=PreStimVASst
  Constant6 : Constant  Value=PreStimBFSHst
  Constant7 : Constant  Value=PreStimGASst
  Constant8 : Constant  Value=PreStimTAst
  Constant9 : Constant  Value=PreStimSOLst
  Demux4 : Demux
  Demux7 : Demux  Outputs=2
  Gain : Gain  Gain=-1
  Mux : Mux  Inputs=9
  Mux1 : Mux  Inputs=3
  Mux2 : Mux  Inputs=3
  Mux3 : Mux  Inputs=3
  Mux4 : Mux
  Sum1 : Sum  Inputs=-+|  SaturateOnIntegerOverflow=on  InputSameDT=on  OutDataTypeStr=Inherit: Same as first input
  Sum11 : Sum  SaturateOnIntegerOverflow=on  InputSameDT=on  OutDataTypeStr=Inherit: Same as first input
  Sum2 : Sum  Inputs=--  SaturateOnIntegerOverflow=on  InputSameDT=on  OutDataTypeStr=Inherit: Same as first input
  Sum3 : Sum  Inputs=-|+  SaturateOnIntegerOverflow=on  InputSameDT=on  OutDataTypeStr=Inherit: Same as first input
  Sum4 : Sum  Inputs=+-|  SaturateOnIntegerOverflow=on  InputSameDT=on  OutDataTypeStr=Inherit: Same as first input
  Sum5 : Sum  Inputs=-+|  SaturateOnIntegerOverflow=on  InputSameDT=on  OutDataTypeStr=Inherit: Same as first input
  Sum6 : Sum  Inputs=-+  SaturateOnIntegerOverflow=on  InputSameDT=on  OutDataTypeStr=Inherit: Same as first input
  Sum7 : Sum  SaturateOnIntegerOverflow=on  InputSameDT=on  OutDataTypeStr=Inherit: Same as first input
  Sum8 : Sum  SaturateOnIntegerOverflow=on  InputSameDT=on  OutDataTypeStr=Inherit: Same as first input
  positive half{1..6} (6 alike) : Saturate  UpperLimit=inf  LowerLimit=0  ZeroCross=off
  Prestimulation : Outport  OutputWhenDisabled=reset  InitialOutput=0  VectorParamsAs1DForOutWhenUnconnected=on
  S_M1 [GLU VAS SOL] : Outport  Port=2  OutputWhenDisabled=reset  InitialOutput=0  VectorParamsAs1DForOutWhenUnconnected=on
  S_M2 [HAM VAS BFSH GAS] : Outport  Port=3  OutputWhenDisabled=reset  InitialOutput=0  VectorParamsAs1DForOutWhenUnconnected=on
  S_M3 [HFL GLU HAM] : Outport  Port=4  OutputWhenDisabled=reset  InitialOutput=0  VectorParamsAs1DForOutWhenUnconnected=on
  S_M4 [HFL GLU HAM] : Outport  Port=5  OutputWhenDisabled=reset  InitialOutput=0  VectorParamsAs1DForOutWhenUnconnected=on
  S_M5 [TA] : Outport  Port=6  OutputWhenDisabled=reset  InitialOutput=0  VectorParamsAs1DForOutWhenUnconnected=on
  wires:
  Sum11/1 -> " 19"/1, Mux3/2  "GLU"
  Sum7/1 -> Mux3/1  "HFL"
  Demux4/4 -> " 18"/1  "Stim_CRF"
  Demux4/3 -> " 16"/1  "Stim_CHAM"
  Mux3/1 -> S_M4 [HFL GLU HAM]/1
  Demux4/2 -> " 15"/1  "Stim_CGLU"
  Demux4/1 -> " 17"/1  "Stim_CHFL"
  Contra Hip swing stimulation/1 -> Demux4/1
  positive half6/1 -> Mux1/3  "HAM"
  positive half2/1 -> Mux1/2  "GLU"
  positive half1/1 -> Mux1/1  "HFL"
  Constant13/1 -> Sum1/1
  " 14"/1 -> positive half6/1  "HAM"
  Mux1/1 -> S_M3 [HFL GLU HAM]/1
  Sum8/1 -> " 14"/1, positive half2/1  "GLU"
  Sum2/1 -> positive half1/1  "HFL"
  " 13"/1 -> Sum8/2
  " 12"/1 -> Sum8/1
  " 11"/1 -> Sum2/2
  " 10"/1 -> Sum2/1
  Sum1/1 -> " 10"/1, " 12"/1
  Demux7/2 -> " 11"/1, " 13"/1  "dphi"
  Demux7/1 -> Sum1/2  "phi"
  phiANDdphiHAT [rad rad/s]/1 -> Demux7/1
  Mux4/1 -> S_M2 [HAM VAS BFSH GAS]/1
  LceTA/1 -> Sum5/2
  Sum6/1 -> S_M5 [TA]/1  "TA"
  " 8"/1 -> Sum6/1
  positive half5/1 -> " 9"/1  "L TA"
  Sum5/1 -> positive half5/1
  LceBFSH/1 -> Sum3/2, Sum4/1
  Sum4/1 -> positive half4/1
  Gain/1 -> Mux4/2  "VAS"
  FmHAM/1 -> " 4"/1  "FmHAM"
  FmGAS/1 -> " 7"/1  "FmGAS"
  positive half4/1 -> " 6"/1  "L BFSH"
  positive half3/1 -> " 5"/1  "L BFSH"
  Sum3/1 -> positive half3/1
  Mux2/1 -> S_M1 [GLU VAS SOL]/1
  FmGLU/1 -> " 3"/1  "FmGLU"
  FmVAS/1 -> " 1"/1  "FmVAS"
  FmSOL/1 -> " 8"/1, " 2"/1  "FmSOL"
  Constant4/1 -> Mux/1
  Constant1/1 -> Mux/2
  Constant2/1 -> Mux/3
  Constant3/1 -> Mux/4
  Constant5/1 -> Mux/5
  Constant6/1 -> Mux/6
  Constant7/1 -> Mux/7
  Constant8/1 -> Mux/9
  Constant9/1 -> Mux/8
  Mux/1 -> Prestimulation/1
  " 3"/1 -> Mux2/1  "GLU"
  " 1"/1 -> Mux2/2  "VAS"
  " 2"/1 -> Mux2/3  "SOL"
  " 4"/1 -> Mux4/1  "HAM"
  Constant10/1 -> Sum3/1
  " 5"/1 -> Gain/1
  Constant11/1 -> Sum4/2
  " 6"/1 -> Mux4/3  "BFSH"
  " 7"/1 -> Mux4/4  "GAS"
  Constant12/1 -> Sum5/1
  " 9"/1 -> Sum6/2
  " 19"/1 -> Mux3/3  "HAM"
  " 15"/1 -> Sum7/1  "HFL"
  " 16"/1 -> Sum7/2  "HFL"
  " 17"/1 -> Sum11/1  "GLU"
  " 18"/1 -> Sum11/2  "GLU"

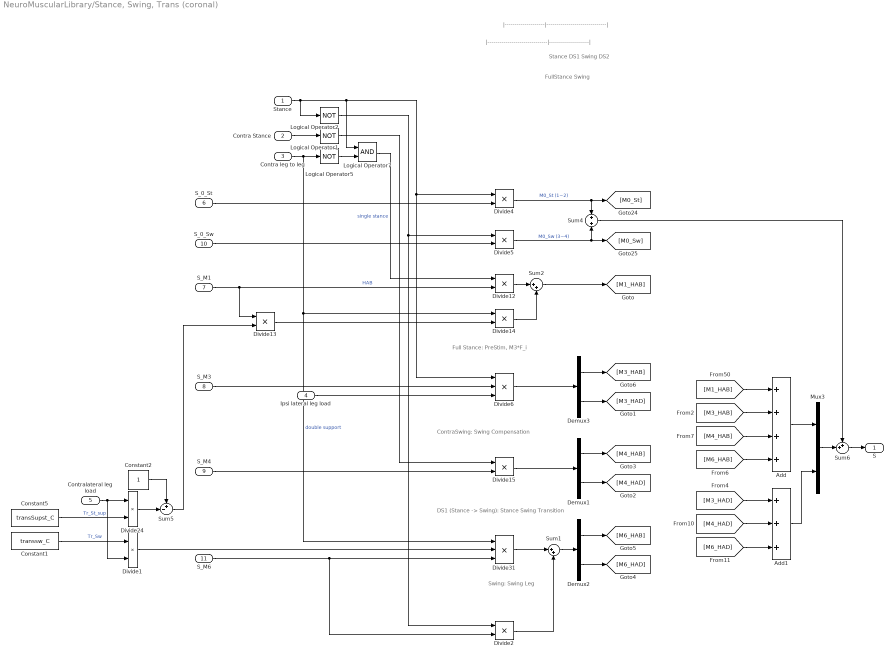
== system NeuroMuscularLibrary/Stance, Swing, Trans (coronal) ==
  note: DS1 (Stance -> Swing):
      | Stance Swing Transition
  note: Swing:
      | Swing Leg
  note: Full Stance:
      | PreStim, M3*F_i
  note: Stance DS1 Swing DS2
  note: FullStance Swing
  note: |------------------------------|--------------------|
  note: |--------------------|------------------------------|
  note: ContraSwing:
      | Swing Compensation
  Stance : Inport
  Contra Stance : Inport  Port=2
  Contra leg to leg : Inport  Port=3
  Ipsi lateral leg load : Inport  Port=4
  Contralateral leg load : Inport  Port=5
  S_0_St : Inport  Port=6
  S_M1 : Inport  Port=7
  S_M3 : Inport  Port=8
  S_M4 : Inport  Port=9
  S_0_Sw : Inport  Port=10
  S_M6 : Inport  Port=11
  Add : Sum  Inputs=4
  Add1 : Sum  Inputs=3
  Constant1 : Constant  Value=transsw_C
  Constant2 : Constant
  Constant5 : Constant  Value=transSupst_C
  Demux1 : Demux  Outputs=2
  Demux2 : Demux  Outputs=2
  Demux3 : Demux  Outputs=2
  Divide{1..2,4..5,12..15,24} (9 alike) : Product
  Divide31 : Product  Inputs=3
  Divide6 : Product  Inputs=3
  Logical Operator1 : Logic  Operator=NOT  AllPortsSameDT=off  OutDataTypeStr=boolean
  Logical Operator2 : Logic  Operator=NOT  AllPortsSameDT=off  OutDataTypeStr=boolean
  Logical Operator5 : Logic  Operator=NOT  AllPortsSameDT=off  OutDataTypeStr=boolean
  Logical Operator7 : Logic  AllPortsSameDT=off  OutDataTypeStr=boolean
  Mux3 : Mux  Inputs=2
  Sum1 : Sum  Inputs=|++  SaturateOnIntegerOverflow=on  InputSameDT=on  OutDataTypeStr=Inherit: Same as first input
  Sum2 : Sum  Inputs=|++  SaturateOnIntegerOverflow=on  InputSameDT=on  OutDataTypeStr=Inherit: Same as first input
  Sum4 : Sum  SaturateOnIntegerOverflow=on  InputSameDT=on  OutDataTypeStr=Inherit: Same as first input
  Sum5 : Sum  Inputs=+-|  SaturateOnIntegerOverflow=on  InputSameDT=on  OutDataTypeStr=Inherit: Same as first input
  Sum6 : Sum  Inputs=++|  SaturateOnIntegerOverflow=on  InputSameDT=on  OutDataTypeStr=Inherit: Same as first input
  S : Outport  OutputWhenDisabled=reset  InitialOutput=0  VectorParamsAs1DForOutWhenUnconnected=on
  wires:
  Contra Stance/1 -> Logical Operator1/1
  S_M4/1 -> Divide15/2
  Logical Operator1/1 -> Divide15/1
  Contralateral leg load/1 -> Divide1/2, Divide24/1
  Divide1/1 -> Divide31/2
  Contra leg to leg/1 -> Logical Operator5/1, Divide31/1, Divide14/1  "double support"
  Stance/1 -> Logical Operator2/1, Divide6/1, Divide4/1, Logical Operator7/1
  Logical Operator2/1 -> Divide2/1, Divide5/1
  Add/1 -> Mux3/1
  Add1/1 -> Mux3/2
  S_M3/1 -> Divide6/2
  Ipsi lateral leg load/1 -> Divide6/3
  S_0_St/1 -> Divide4/2
  S_0_Sw/1 -> Divide5/2
  Mux3/1 -> Sum6/2
  Sum6/1 -> S/1
  S_M6/1 -> Divide31/3, Divide2/2
  Divide4/1 -> Sum4/1, [M0_St]  "M0_St (1~2)"
  Divide5/1 -> Sum4/2, [M0_Sw]  "M0_Sw (3~4)"
  Divide31/1 -> Sum1/1
  Divide2/1 -> Sum1/2
  S_M1/1 -> Divide12/2, Divide13/1  "HAB"
  Divide12/1 -> Sum2/1
  Divide13/1 -> Divide14/2
  Divide14/1 -> Sum2/2
  Logical Operator5/1 -> Logical Operator7/2
  Logical Operator7/1 -> Divide12/1  "single stance"
  Divide24/1 -> Sum5/2
  Constant2/1 -> Sum5/1
  Sum5/1 -> Divide13/2
  Constant5/1 -> Divide24/2  "Tr_St_sup"
  Constant1/1 -> Divide1/1  "Tr_Sw"
  Sum2/1 -> [M1_HAB]
  Divide6/1 -> Demux3/1
  Demux3/1 -> [M3_HAB]
  Demux3/2 -> [M3_HAD]
  Divide15/1 -> Demux1/1
  Demux1/1 -> [M4_HAB]
  Demux1/2 -> [M4_HAD]
  Demux2/1 -> [M6_HAB]
  Demux2/2 -> [M6_HAD]
  Sum1/1 -> Demux2/1
  Sum4/1 -> Sum6/1
  [M1_HAB] -> Add/1
  [M3_HAB] -> Add/2
  [M3_HAD] -> Add1/1
  [M4_HAB] -> Add/3
  [M6_HAB] -> Add/4
  [M4_HAD] -> Add1/2
  [M6_HAD] -> Add1/3
